simulink model "hw3_2c_CoupledNeuralOscillator"  (R2013a)
settings: Solver=ode45  StartTime=0.0  StopTime=30  RelTol=1e-3
InitFcn:
  | % CPG parameters
  | x0 = 5;
  | 
  | % tau_prime > tau because the auto-adaptation decay takes longer to occur. must also meet the quadratic difference condition
  | tau_x = 1; % [s]
  | tau_a = 12; % [s]
  | 
  | xth = 0; % percent
  | 
  | wp = 2.5; % [dimensionless]
settings Model: Creator=benshih  LastModifiedBy=benshih

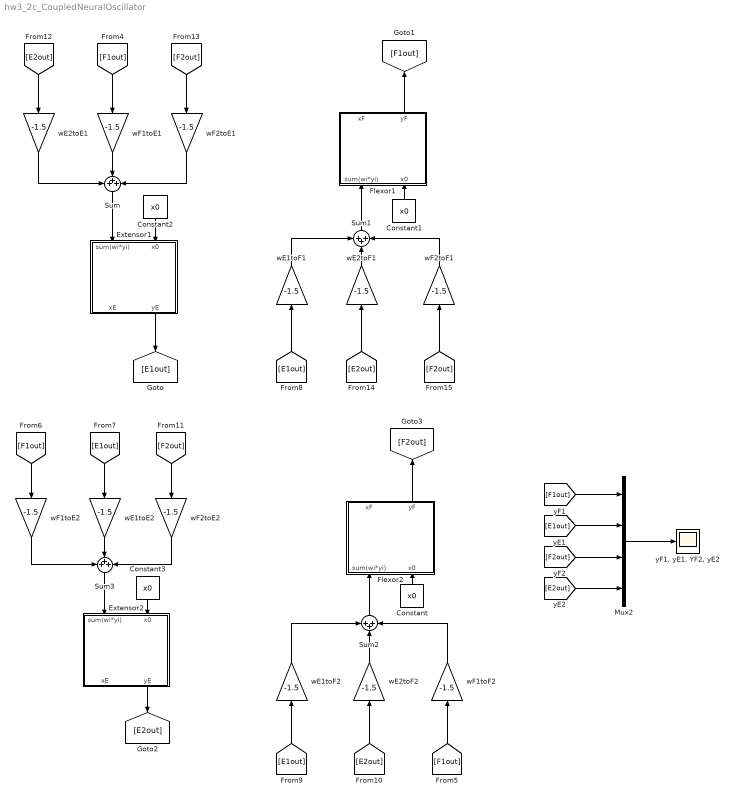
== system hw3_2c_CoupledNeuralOscillator ==
  Constant{,1..3} (4 alike) : Constant  Value=x0
  Extensor1 : Subsystem
  Extensor2 : Subsystem
  Flexor1 : Subsystem
  Flexor2 : Subsystem
  Mux2 : Mux
  Sum{,1..3} (4 alike) : Sum  Inputs=+++
  wE1toE2 : Gain  Gain=-1.5
  wE1toF1 : Gain  Gain=-1.5
  wE1toF2 : Gain  Gain=-1.5
  wE2toE1 : Gain  Gain=-1.5
  wE2toF1 : Gain  Gain=-1.5
  wE2toF2 : Gain  Gain=-1.5
  wF1toE1 : Gain  Gain=-1.5
  wF1toE2 : Gain  Gain=-1.5
  wF1toF2 : Gain  Gain=-1.5
  wF2toE1 : Gain  Gain=-1.5
  wF2toE2 : Gain  Gain=-1.5
  wF2toF1 : Gain  Gain=-1.5
  "yF1, yE1, YF2, yE2" : Scope
      settings: ShowLegends=on  TimeRange=10  YMin=0.2999985  YMax=0.3000015  SaveName=ScopeData2
  wires:
  Constant/1 -> Flexor2/2(x0)
  wF1toE1/1 -> Sum/2
  Sum/1 -> Extensor1/1(sum(wi*yi))
  Sum3/1 -> Extensor2/1(sum(wi*yi))
  wE1toE2/1 -> Sum3/2
  Sum1/1 -> Flexor1/1(sum(wi*yi))
  wE2toF1/1 -> Sum1/2
  Sum2/1 -> Flexor2/1(sum(wi*yi))
  wE2toF2/1 -> Sum2/2
  Extensor1/2(yE) -> [E1out]
  Flexor1/2(yF) -> [F1out]
  wE1toF1/1 -> Sum1/1
  Constant1/1 -> Flexor1/2(x0)
  Constant2/1 -> Extensor1/2(x0)
  wE2toE1/1 -> Sum/1
  wF2toE1/1 -> Sum/3
  wF2toF1/1 -> Sum1/3
  Constant3/1 -> Extensor2/2(x0)
  wF2toE2/1 -> Sum3/3
  wF1toE2/1 -> Sum3/1
  wF1toF2/1 -> Sum2/3
  wE1toF2/1 -> Sum2/1
  Extensor2/2(yE) -> [E2out]
  Mux2/1 -> "yF1, yE1, YF2, yE2"/1
  [E2out] -> Mux2/4
  [F2out] -> Mux2/3
  Flexor2/2(yF) -> [F2out]
  [F1out] -> wF1toE1/1
  [F1out] -> wF1toF2/1
  [F1out] -> wF1toE2/1
  [E1out] -> wE1toE2/1
  [E1out] -> wE1toF1/1
  [E1out] -> wE1toF2/1
  [E2out] -> wE2toF2/1
  [F2out] -> wF2toE2/1
  [F2out] -> wF2toE1/1
  [E2out] -> wE2toE1/1
  [E2out] -> wE2toF1/1
  [F2out] -> wF2toF1/1
  [E1out] -> Mux2/2
  [F1out] -> Mux2/1

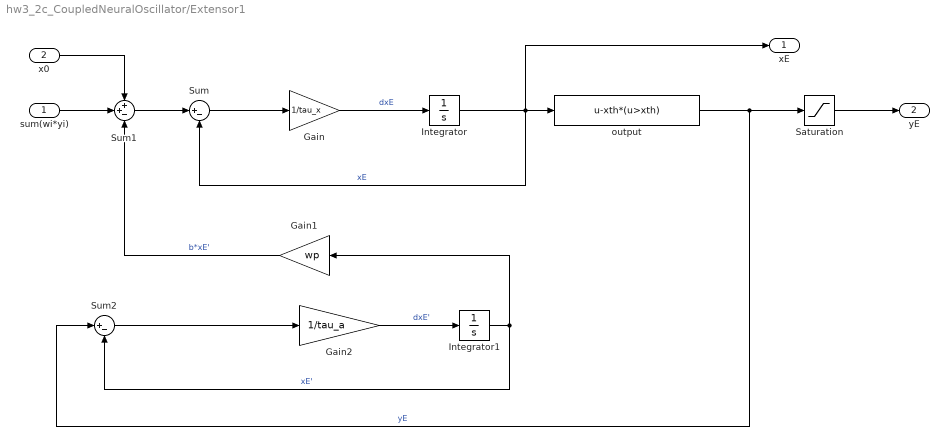
== system hw3_2c_CoupledNeuralOscillator/Extensor1 ==
  sum(wi*yi) : Inport
  x0 : Inport  Port=2
  Gain : Gain  Gain=1/tau_x
  Gain1 : Gain  Gain=wp
  Gain2 : Gain  Gain=1/tau_a
  Integrator : Integrator  InitialCondition=1
  Integrator1 : Integrator
  Saturation : Saturate  UpperLimit=Inf  LowerLimit=0
  Sum : Sum  Inputs=|+-
  Sum1 : Sum  Inputs=++-
  Sum2 : Sum  Inputs=|+-
  output : Fcn  Expr=u-xth*(u>xth)
  xE : Outport
  yE : Outport  Port=2
  wires:
  Integrator/1 -> xE/1, Sum/2, output/1  "xE"
  Sum/1 -> Gain/1
  Gain/1 -> Integrator/1  "dxE"
  output/1 -> Sum2/1, Saturation/1  "yE"
  Sum1/1 -> Sum/1
  sum(wi*yi)/1 -> Sum1/2
  Gain1/1 -> Sum1/3  "b*xE'"
  Gain2/1 -> Integrator1/1  "dxE'"
  Integrator1/1 -> Gain1/1, Sum2/2  "xE'"
  Sum2/1 -> Gain2/1
  x0/1 -> Sum1/1
  Saturation/1 -> yE/1

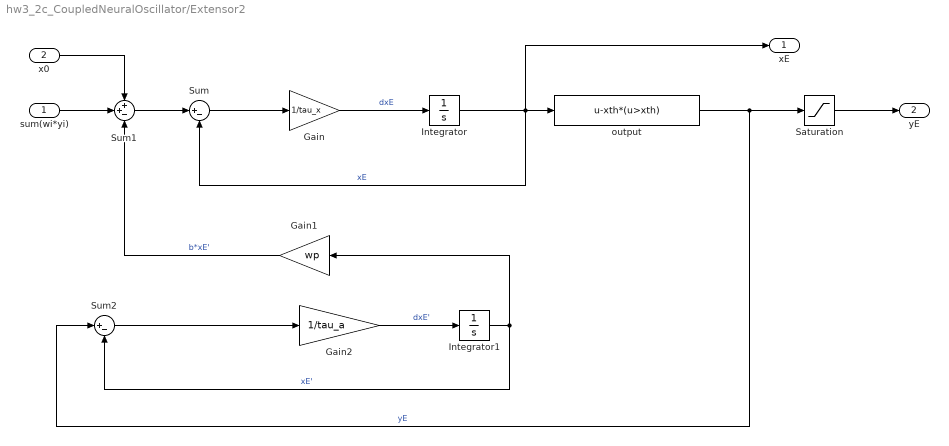
== system hw3_2c_CoupledNeuralOscillator/Extensor2 ==
  sum(wi*yi) : Inport
  x0 : Inport  Port=2
  Gain : Gain  Gain=1/tau_x
  Gain1 : Gain  Gain=wp
  Gain2 : Gain  Gain=1/tau_a
  Integrator : Integrator  InitialCondition=1
  Integrator1 : Integrator
  Saturation : Saturate  UpperLimit=Inf  LowerLimit=0
  Sum : Sum  Inputs=|+-
  Sum1 : Sum  Inputs=++-
  Sum2 : Sum  Inputs=|+-
  output : Fcn  Expr=u-xth*(u>xth)
  xE : Outport
  yE : Outport  Port=2
  wires:
  Integrator/1 -> xE/1, Sum/2, output/1  "xE"
  Sum/1 -> Gain/1
  Gain/1 -> Integrator/1  "dxE"
  output/1 -> Sum2/1, Saturation/1  "yE"
  Sum1/1 -> Sum/1
  sum(wi*yi)/1 -> Sum1/2
  Gain1/1 -> Sum1/3  "b*xE'"
  Gain2/1 -> Integrator1/1  "dxE'"
  Integrator1/1 -> Gain1/1, Sum2/2  "xE'"
  Sum2/1 -> Gain2/1
  x0/1 -> Sum1/1
  Saturation/1 -> yE/1

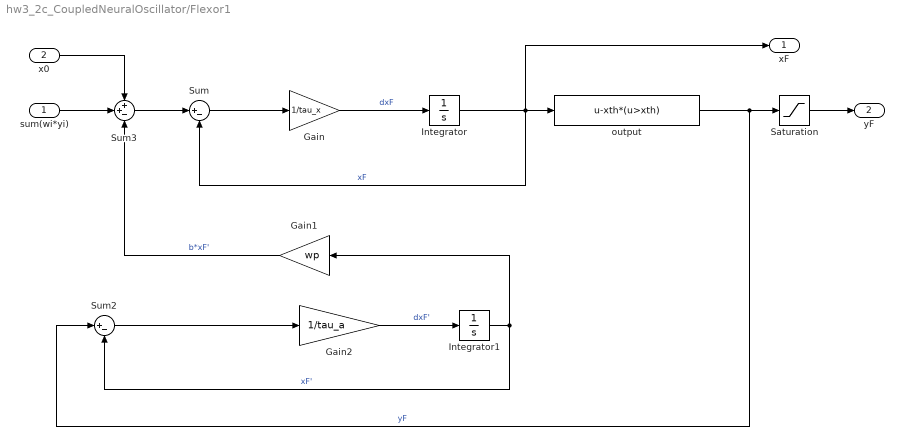
== system hw3_2c_CoupledNeuralOscillator/Flexor1 ==
  sum(wi*yi) : Inport
  x0 : Inport  Port=2
  Gain : Gain  Gain=1/tau_x
  Gain1 : Gain  Gain=wp
  Gain2 : Gain  Gain=1/tau_a
  Integrator : Integrator
  Integrator1 : Integrator
  Saturation : Saturate  UpperLimit=Inf  LowerLimit=0
  Sum : Sum  Inputs=|+-
  Sum2 : Sum  Inputs=|+-
  Sum3 : Sum  Inputs=++-
  output : Fcn  Expr=u-xth*(u>xth)
  xF : Outport
  yF : Outport  Port=2
  wires:
  Sum2/1 -> Gain2/1
  Integrator1/1 -> Sum2/2, Gain1/1  "xF'"
  Gain2/1 -> Integrator1/1  "dxF'"
  Gain1/1 -> Sum3/3  "b*xF'"
  Sum3/1 -> Sum/1
  output/1 -> Saturation/1, Sum2/1  "yF"
  Gain/1 -> Integrator/1  "dxF"
  Sum/1 -> Gain/1
  Integrator/1 -> output/1, Sum/2, xF/1  "xF"
  sum(wi*yi)/1 -> Sum3/2
  x0/1 -> Sum3/1
  Saturation/1 -> yF/1

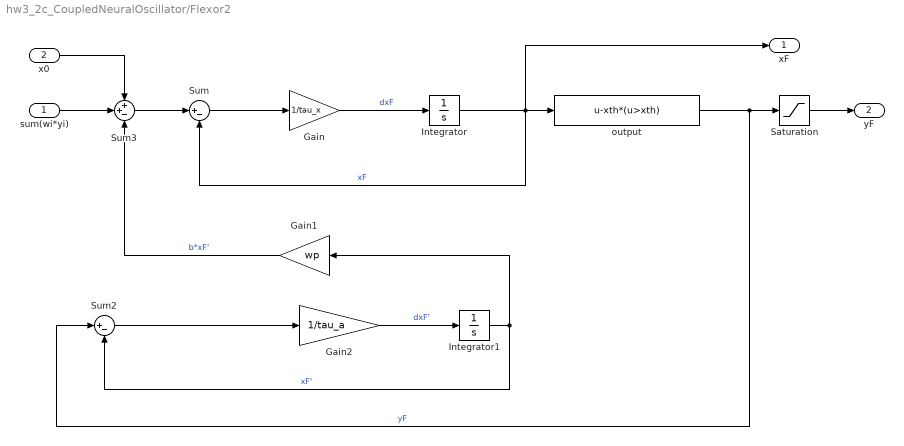
== system hw3_2c_CoupledNeuralOscillator/Flexor2 ==
  sum(wi*yi) : Inport
  x0 : Inport  Port=2
  Gain : Gain  Gain=1/tau_x
  Gain1 : Gain  Gain=wp
  Gain2 : Gain  Gain=1/tau_a
  Integrator : Integrator
  Integrator1 : Integrator
  Saturation : Saturate  UpperLimit=Inf  LowerLimit=0
  Sum : Sum  Inputs=|+-
  Sum2 : Sum  Inputs=|+-
  Sum3 : Sum  Inputs=++-
  output : Fcn  Expr=u-xth*(u>xth)
  xF : Outport
  yF : Outport  Port=2
  wires:
  Sum2/1 -> Gain2/1
  Integrator1/1 -> Sum2/2, Gain1/1  "xF'"
  Gain2/1 -> Integrator1/1  "dxF'"
  Gain1/1 -> Sum3/3  "b*xF'"
  Sum3/1 -> Sum/1
  output/1 -> Saturation/1, Sum2/1  "yF"
  Gain/1 -> Integrator/1  "dxF"
  Sum/1 -> Gain/1
  Integrator/1 -> output/1, Sum/2, xF/1  "xF"
  sum(wi*yi)/1 -> Sum3/2
  x0/1 -> Sum3/1
  Saturation/1 -> yF/1
